simulink model "UKF_liuxg"  (R2017a)
settings: Solver=FixedStepAuto  StartTime=0.0  StopTime=13135  FixedStep=1  RelTol=1e-3
undefined symbols (not defined in the file): sigbuilder_block
libraries: dspmtrx3 x2
settings Model: Creator=HP  LastModifiedBy=HP
settings DataIOCC: ReturnWorkspaceOutputs=on
settings DebuggingCC: UnconnectedInputMsg=none  UnconnectedOutputMsg=none  UnconnectedLineMsg=none
settings ModelReferenceCC: EnableRefExpFcnMdlSchedulingChecks=off
settings SFSimCC: SimUseLocalCustomCode=on
settings RTWCC: RTWUseLocalCustomCode=on

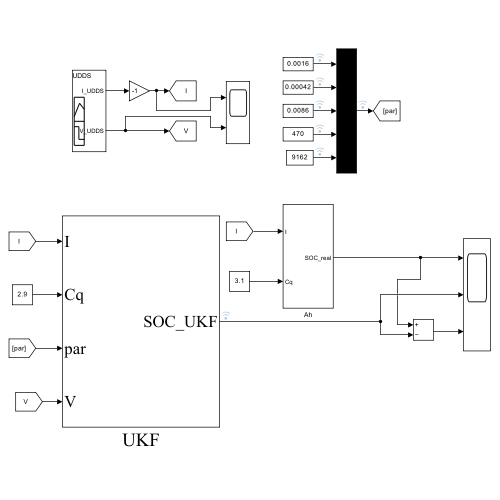
[thumbnail: Simulink's stored preview of the top-level diagram]
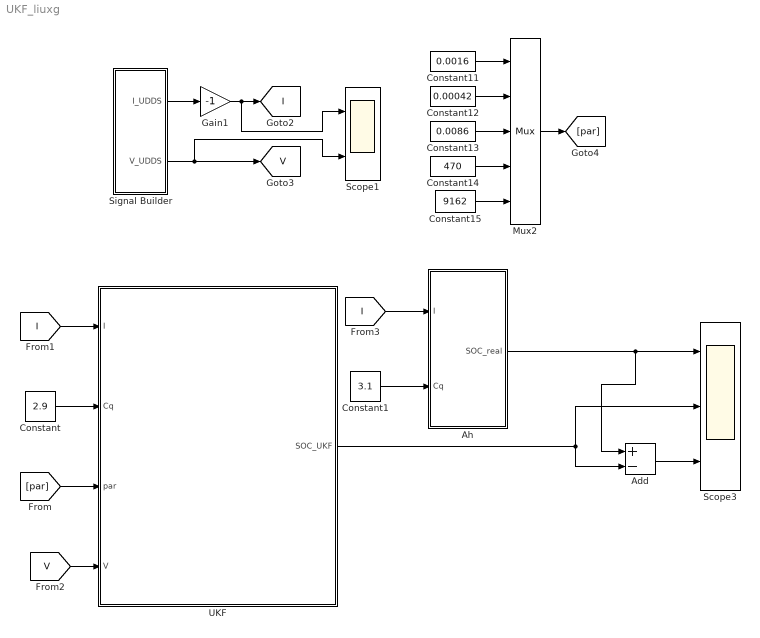
== system UKF_liuxg ==
  Add : Sum  Inputs=+-
  Ah : Subsystem
  Constant : Constant  Value=2.9
  Constant1 : Constant  Value=3.1
  Constant11 : Constant  Value=0.0016
  Constant12 : Constant  Value=0.00042
  Constant13 : Constant  Value=0.0086
  Constant14 : Constant  Value=470
  Constant15 : Constant  Value=9162
  Gain1 : Gain  Gain=-1
  Mux2 : Mux  Inputs=5
  Scope1 : Scope  NumInputPorts=2
  Scope3 : Scope  NumInputPorts=3
  Signal Builder : Subsystem  Tag=STV Subsys  LoadFcn=sigbuilder_block('load');  StartFcn=sigbuilder_block('start');  StopFcn=sigbuilder_block('stop');  ClipboardFcn=sigbuilder_block('clipboard');  mask(Sigbuilder block){tuvar=[0:10]}
      mask init:
      | if ~strcmp(get_param(bdroot(gcb),'SimulationStatus'),'stopped'),tuvar = sigbuilder_block('maskInit'); end
      settings: CopyFcn=sigbuilder_block('copy');  DeleteFcn=sigbuilder_block('delete');  ModelCloseFcn=sigbuilder_block('modelClose');  PreSaveFcn=sigbuilder_block('preSave');  PauseFcn=sigbuilder_block('pause');  ContinueFcn=sigbuilder_block('continue');  NameChangeFcn=sigbuilder_block('namechange');  OpenFcn=sigbuilder_block('open',[0 63 1141.2 523.8 ]);  CloseFcn=sigbuilder_block('close');
      mask Display: plot(0, 0, 100, 100,[2, 2, 32, 32, 2], [68, 8, 8, 68, 68],[32, 2], [38, 38], [32, 19, 2],[53, 60, 44], [32, 17, 17, 2],[16, 16, 31, 31]);txt = getActiveGroup(gcbh);text(2, 100, txt,'verticalAlignment', 'top');
  UKF : Subsystem  mask{Q_UKF=[0.0000000001,0.00001,0.00000001], R_UKF=0.1, X0_UKF=[0.8;0;0], P0_UKF=[0.01,0.01,0.01], f_OCV=[-542.328042776627	3066.57848545083	-7520.83333797876	10535.7804287577	-9327.72222618654	5441.66203885271	-2111.60737486106	536.514433511755	-85.4036277861597	8.01612301618486	2.03460000000008], beta=2, alf=1, ki=0, L=3}
      mask prompts: Q_UKF "系统协方差Q"; R_UKF "测量协方差R"; X0_UKF "状态初始值X0"; P0_UKF "估计协方差初始值P0"; f_OCV "开路电压对SOC的函数"; beta "非负权系数beta"; alf "采样点分布状态参数alf"; ki "无界非待选参数ki"; L "状态维度L"
      mask DialogControl DescGroupVar Prompt: UKF滤波算法
      mask DialogControl ParameterGroupVar Prompt: 滤波参数设置
      mask DialogControl ParameterGroupVar2 Prompt: sigma参数设置
  tag scope: I=global, V=global
  wires:
  Constant15/1 -> Mux2/5
  Constant11/1 -> Mux2/1
  Constant13/1 -> Mux2/3
  Constant14/1 -> Mux2/4
  Constant12/1 -> Mux2/2
  Mux2/1 -> [par]
  Signal Builder/1(I_UDDS) -> Gain1/1
  Signal Builder/2(V_UDDS) -> [V], Scope1/2
  Gain1/1 -> Scope1/1, [I]
  [par] -> UKF/3(par)
  [I] -> UKF/1(I)
  [V] -> UKF/4(V)
  Constant/1 -> UKF/2(Cq)
  UKF/1(SOC_UKF) -> Scope3/2, Add/2
  [I] -> Ah/1(I)
  Constant1/1 -> Ah/2(Cq)
  Ah/1(SOC_real) -> Add/1, Scope3/1
  Add/1 -> Scope3/3

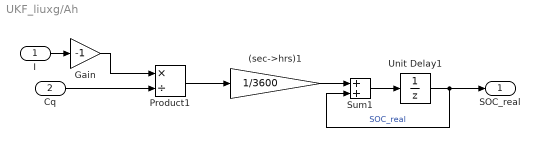
== system UKF_liuxg/Ah ==
  I : Inport
  Cq : Inport  Port=2
  (sec->hrs)1 : Gain  Gain=1/3600  SaturateOnIntegerOverflow=on  OutDataTypeStr=Inherit: Same as input  ParamDataTypeStr=Inherit: Same as input
  Gain : Gain  Gain=-1
  Product1 : Product  Inputs=*/
  Sum1 : Sum
  Unit Delay1 : UnitDelay  InitialCondition=1  SampleTime=-1  HasFrameUpgradeWarning=on
  SOC_real : Outport
  wires:
  I/1 -> Gain/1
  Gain/1 -> Product1/1
  Product1/1 -> (sec->hrs)1/1
  (sec->hrs)1/1 -> Sum1/1
  Unit Delay1/1 -> Sum1/2, SOC_real/1  "SOC_real"
  Sum1/1 -> Unit Delay1/1
  Cq/1 -> Product1/2

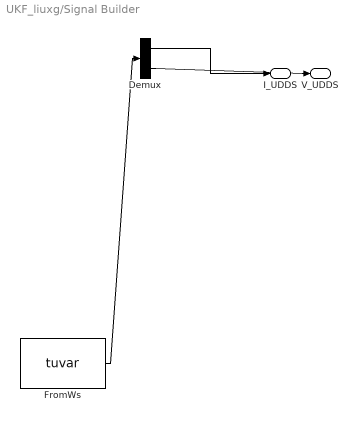
== system UKF_liuxg/Signal Builder ==
  Demux : Demux  Tag=STV Demux  Outputs=2
  FromWs : FromWorkspace  Tag=STV FromWs  VariableName=tuvar
      SigBuilderData=|
      | dataSet.timeRange = [1 13135]
      | dataSet.name = 'UDDS'
      | sbobj.Name = 'Signal Builder'
      | sbobj.Groups.Name = 'UDDS'
      | sbobj.Groups.Signals(1).Name = 'I_UDDS'
      | sbobj.Groups.Signals(1).XData = [1 2 3 4 5 6 7 8 9 10 11 12 ... (13135 elements, 1x13135)]
      | sbobj.Groups.Signals(1).YData = [0 -0.0248 -0.1178 -0.1178 -0.1178 -0.1178 -0.1178 -0.1178 -0.1178 -0.1178 -0.1178 -0.1178 ... (13135 elements, 1x13135)]
      | sbobj.Groups.Signals(2).Name = 'V_UDDS'
      | sbobj.Groups.Signals(2).XData = [1 2 3 4 5 6 7 8 9 10 11 12 ... (13135 elements, 1x13135)]
      | sbobj.Groups.Signals(2).YData = [2.6686 2.6686 2.6683 2.6683 2.6683 2.6677 2.6677 2.6677 2.6677 2.6674 2.6674 2.6674 ... (13135 elements, 1x13135)]
      | sbobj.Groups.TimeRange = [1 9002]
  I_UDDS : Outport  Tag=STV Outport
  V_UDDS : Outport  Tag=STV Outport  Port=2
  wires:
  FromWs/1 -> Demux/1
  Demux/1 -> I_UDDS/1
  Demux/2 -> V_UDDS/1

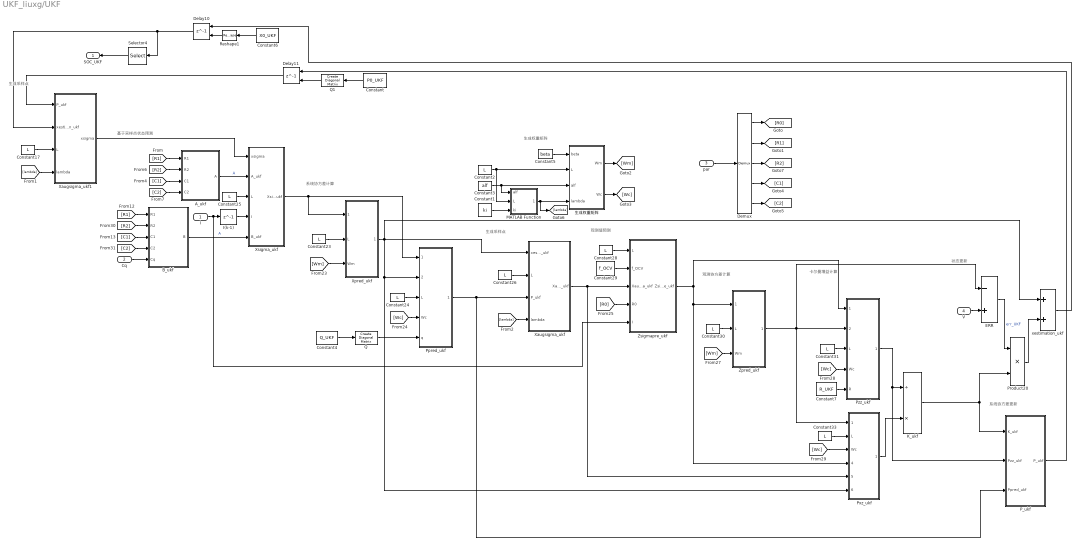
== system UKF_liuxg/UKF ==
  note: 生成权重矩阵
  note: 系统协方差更新
  note: 状态更新
  note: 卡尔曼增益计算
  note: 观测协方差计算
  note: 观测值预测
  note: 生成采样点
  note: 系统协方差计算
  note: 基于采样点状态预测
  note: 生成采样点
  I : Inport
  Cq : Inport  Port=2
  par : Inport  Port=3
  V : Inport  Port=4
  A_ukf : MATLAB Function  TreatAsAtomicUnit=on
  B_ukf : MATLAB Function  TreatAsAtomicUnit=on
  Constant : Constant  Value=P0_UKF
  Constant1 : Constant  Value=ki
  Constant{2,17,23..26,28,30..31,33} (10 alike) : Constant  Value=L
  Constant29 : Constant  Value=f_OCV
  Constant3 : Constant  Value=alf
  Constant4 : Constant  Value=Q_UKF
  Constant5 : Constant  Value=beta
  Constant6 : Constant  Value=X0_UKF
  Constant7 : Constant  Value=R_UKF
  Delay10 : Delay  DelayLength=1  InitialConditionSource=Input port
      settings: InputPortMap=u0,p4
  Delay11 : Delay  DelayLength=1  InitialConditionSource=Input port  InitialCondition=0.001*eye(L)
      settings: InputPortMap=u0,p4
  Demux : Demux  Outputs=5
  ERR : Sum  Inputs=-+
  I(k-1) : Delay  DelayLength=1
  K_ukf : Product  Inputs=/*
  MATLAB Function : MATLAB Function  TreatAsAtomicUnit=on
  P_ukf : MATLAB Function  TreatAsAtomicUnit=on
  Ppred_ukf : MATLAB Function  TreatAsAtomicUnit=on
  Product20 : Product
  Pxz_ukf : MATLAB Function  TreatAsAtomicUnit=on
  Pzz_ukf : MATLAB Function  TreatAsAtomicUnit=on
  Q : dspmtrx3/Create Diagonal Matrix
  Q1 : dspmtrx3/Create Diagonal Matrix
  Reshape1 : Reshape  OutputDimensionality=Customize  OutputDimensions=[3,1]
  Selector4 : Selector  NumberOfDimensions=2  InputPortWidth=3  IndexOptions=Index vector (dialog),Index vector (dialog)  Indices=[1],1  OutputSizes=1,1
  Xaugsigma_ukf : MATLAB Function  TreatAsAtomicUnit=on
  Xaugsigma_ukf1 : MATLAB Function  TreatAsAtomicUnit=on
  Xpred_ukf : MATLAB Function  TreatAsAtomicUnit=on
  Xsigma_ukf : MATLAB Function  TreatAsAtomicUnit=on
  Zpred_ukf : MATLAB Function  TreatAsAtomicUnit=on
  Zsigmapre_ukf : MATLAB Function  TreatAsAtomicUnit=on
  xestimation_ukf : Sum
  生成权重矩阵 : MATLAB Function  TreatAsAtomicUnit=on
  SOC_UKF : Outport
  wires:
  Reshape1/1 -> Delay10/2
  [R0] -> Zsigmapre_ukf/4(R0)
  Q/1 -> Ppred_ukf/5(q)
  P_ukf/1(P_ukf) -> Delay11/1
  Constant17/1 -> Xaugsigma_ukf1/3(L)
  Zsigmapre_ukf/1(Zsigmapre_ukf) -> Pzz_ukf/1(Zsigmapre_ukf), Zpred_ukf/1(Zsigmapre_ukf), Pxz_ukf/4(Zsigmapre_ukf)
  生成权重矩阵/1(Wm) -> [Wm]
  Constant7/1 -> Pzz_ukf/5(R)
  Constant29/1 -> Zsigmapre_ukf/2(f_OCV)
  Zpred_ukf/1(Zpred_ukf) -> Pzz_ukf/2(Zpred_ukf), Pxz_ukf/1(Zpred_ukf), ERR/1
  Xpred_ukf/1(Xpred_ukf) -> Pxz_ukf/6(Xpred_ukf), Ppred_ukf/2(Xpred_ukf), xestimation_ukf/1, Xaugsigma_ukf/1(xestimation_ukf)
  Xsigma_ukf/1(Xsigma_ukf) -> Xpred_ukf/1(Xsigma_ukf), Ppred_ukf/1(Xsigma_ukf)
  Delay11/1 -> Xaugsigma_ukf1/1(P_ukf)
  Ppred_ukf/1(Ppred_ukf) -> P_ukf/3(Ppred_ukf), Xaugsigma_ukf/3(P_ukf)
  Xaugsigma_ukf1/1(xsigma) -> Xsigma_ukf/1(xsigma)
  xestimation_ukf/1 -> Delay10/1
  I(k-1)/1 -> Xsigma_ukf/4(I)
  B_ukf/1(B) -> Xsigma_ukf/5(B_ukf)  "A"
  Constant26/1 -> Xaugsigma_ukf/2(L)
  [lambda] -> Xaugsigma_ukf/4(lambda)
  Delay10/1 -> Xaugsigma_ukf1/2(xestimation_ukf), Selector4/1
  Xaugsigma_ukf/1(Xaugsigma_ukf) -> Zsigmapre_ukf/3(Xaugsigma_ukf), Pxz_ukf/5(Xaugsigma_ukf)
  [R1] -> B_ukf/1(R1)
  [lambda] -> Xaugsigma_ukf1/4(lambda)
  Constant33/1 -> Pxz_ukf/2(L)
  Constant4/1 -> Q/1
  Constant30/1 -> Zpred_ukf/2(L)
  K_ukf/1 -> Product20/2, P_ukf/1(K_ukf)
  Constant28/1 -> Zsigmapre_ukf/1(L)
  [Wm] -> Xpred_ukf/3(Wm)
  生成权重矩阵/2(Wc) -> [Wc]
  Selector4/1 -> SOC_UKF/1
  [Wc] -> Pxz_ukf/3(Wc)
  Constant31/1 -> Pzz_ukf/3(L)
  [Wm] -> Zpred_ukf/3(Wm)
  Constant6/1 -> Reshape1/1
  A_ukf/1(A) -> Xsigma_ukf/2(A_ukf)  "A"
  Product20/1 -> xestimation_ukf/2
  [Wc] -> Pzz_ukf/4(Wc)
  Pzz_ukf/1(Pzz_ukf) -> K_ukf/1, P_ukf/2(Pzz_ukf)
  [Wc] -> Ppred_ukf/4(Wc)
  Pxz_ukf/1(Pxz_ukf) -> K_ukf/2
  Constant24/1 -> Ppred_ukf/3(L)
  V/1 -> ERR/2
  Constant23/1 -> Xpred_ukf/2(L)
  [C1] -> A_ukf/3(C1)
  Constant25/1 -> Xsigma_ukf/3(L)
  [C2] -> B_ukf/4(C2)
  Cq/1 -> B_ukf/5(Cq)
  [R1] -> A_ukf/1(R1)
  [R2] -> A_ukf/2(R2)
  [C2] -> A_ukf/4(C2)
  I/1 -> Zsigmapre_ukf/5(I), I(k-1)/1
  Demux/4 -> [C1]
  Demux/3 -> [R2]
  Demux/1 -> [R0]
  par/1 -> Demux/1
  Demux/5 -> [C2]
  Demux/2 -> [R1]
  [R2] -> B_ukf/2(R2)
  [C1] -> B_ukf/3(C1)
  Constant/1 -> Q1/1
  Q1/1 -> Delay11/2
  Constant5/1 -> 生成权重矩阵/1(beta)
  Constant2/1 -> 生成权重矩阵/2(L), MATLAB Function/2(L)
  Constant3/1 -> 生成权重矩阵/3(alf), MATLAB Function/1(alf)
  MATLAB Function/1(lambda) -> 生成权重矩阵/4(lambda), [lambda]
  Constant1/1 -> MATLAB Function/3(ki)
  ERR/1 -> Product20/1  "err_UKF"

== matlab function UKF_liuxg/UKF/生成权重矩阵 ==
  data: beta input; L input; alf input; lambda input; Wm output size=[7,1]; Wc output size=[7,1]
function [Wm,Wc] = fcn(beta,L,alf,lambda)
Wm=zeros(7,1);
Wc=zeros(7,1);
Wm(1)=lambda/(L+lambda);
Wc(1)=lambda/((L+lambda)+1-alf^2+beta);
for j=2:2*L+1
    Wm(j)=1/(2*(L+lambda));%下标m为均值权重
    Wc(j)=1/(2*(L+lambda));%下标c为协方差权重
end

== matlab function UKF_liuxg/UKF/Xpred_ukf ==
  data: Xsigma_ukf input; Xpred_ukf output; L input; Wm input
function Xpred_ukf  = E(Xsigma_ukf,L,Wm)
Xpred_ukf=zeros(size(Xsigma_ukf,1),1);
for k=1:2*L+1
    Xpred_ukf=Xpred_ukf+Wm(k)*Xsigma_ukf(:,k);
end
end

== matlab function UKF_liuxg/UKF/Ppred_ukf ==
  data: Xsigma_ukf input; Xpred_ukf input; Ppred_ukf output size=[L,L]; L input; Wc input; q input
function Ppred_ukf  = EAE(Xsigma_ukf,Xpred_ukf,L,Wc,q)
Ppred_ukf=zeros(size(Xsigma_ukf,1),size(Xsigma_ukf,1));%协方差预测均值
for k=1:2*L+1
    Ppred_ukf=Ppred_ukf+Wc(k)*(Xsigma_ukf(:,k)-Xpred_ukf)*(Xsigma_ukf(:,k)-Xpred_ukf)';
end
Ppred_ukf=Ppred_ukf+q;
end

== matlab function UKF_liuxg/UKF/Xaugsigma_ukf ==
  data: xestimation_ukf input; L input; Xaugsigma_ukf output size=[L,2*L+1]; P_ukf input; lambda input
function Xaugsigma_ukf = sigma(xestimation_ukf,L,P_ukf,lambda)
cho_ukf=(chol(P_ukf*(L+lambda)))';%cho=chol(X)用于对矩阵X进行Cholesky分解，产生一个上三角cho，使得cho'cho=X，若X为非对称正定，则报错；
XaugsigmaP1_ukf=zeros(size(xestimation_ukf,1),size(xestimation_ukf,1));
XaugsigmaP2_ukf=zeros(size(xestimation_ukf,1),size(xestimation_ukf,1));
for k=1:L
    XaugsigmaP1_ukf(:,k)=xestimation_ukf+cho_ukf(:,k);
    XaugsigmaP2_ukf(:,k)=xestimation_ukf-cho_ukf(:,k);
end
Xaugsigma_ukf=[xestimation_ukf XaugsigmaP1_ukf XaugsigmaP2_ukf];%获得2*L+1个sigma点
end

== matlab function UKF_liuxg/UKF/Zsigmapre_ukf ==
  data: L input; Zsigmapre_ukf output size=[1,2*L+1]; f_OCV input; Xaugsigma_ukf input; R0 input; I input
function Zsigmapre_ukf= err(L,f_OCV,Xaugsigma_ukf,R0,I)
    Zsigmapre_ukf=zeros(1,2*size(Xaugsigma_ukf,1)+1);
    for k=1:2*L+1
        Zsigmapre_ukf(1,k)=polyval(f_OCV,Xaugsigma_ukf(1,k))-Xaugsigma_ukf(2,k)-Xaugsigma_ukf(3,k)-R0*I;
    end
end

== matlab function UKF_liuxg/UKF/Zpred_ukf ==
  data: Zsigmapre_ukf input; Zpred_ukf output; L input; Wm input
function Zpred_ukf  = E(Zsigmapre_ukf,L,Wm)
Zpred_ukf=zeros(size(Zsigmapre_ukf,1),1);
for k=1:2*L+1
    Zpred_ukf=Zpred_ukf+Wm(k)*Zsigmapre_ukf(:,k);
end
end

== matlab function UKF_liuxg/UKF/Pzz_ukf ==
  data: Zsigmapre_ukf input; Zpred_ukf input; Pzz_ukf output size=[1,1]; L input; Wc input; R input
function Pzz_ukf  = EAE(Zsigmapre_ukf,Zpred_ukf,L,Wc,R)
Pzz_ukf=zeros(size(Zsigmapre_ukf,1),size(Zsigmapre_ukf,1));%协方差预测均值
for k=1:2*L+1
    Pzz_ukf=Pzz_ukf+Wc(k)*(Zsigmapre_ukf(:,k)-Zpred_ukf)*(Zsigmapre_ukf(:,k)-Zpred_ukf)';
end
Pzz_ukf=Pzz_ukf+R;
end

== matlab function UKF_liuxg/UKF/Pxz_ukf ==
  data: Zpred_ukf input; L input; Wc input; Zsigmapre_ukf input; Xaugsigma_ukf input; Xpred_ukf input; Pxz_ukf output size=[L,1]
function Pxz_ukf= fcn(Zpred_ukf,L,Wc,Zsigmapre_ukf,Xaugsigma_ukf,Xpred_ukf)
    Pxz_ukf=zeros(size(Xpred_ukf,1),1);
    for k=1:2*L+1
        Pxz_ukf=Pxz_ukf+Wc(k)*(Xaugsigma_ukf(:,k)-Xpred_ukf)*(Zsigmapre_ukf(1,k)-Zpred_ukf)'; 
    end

== matlab function UKF_liuxg/UKF/Xsigma_ukf ==
  data: xsigma input size=[L,2*L+1]; A_ukf input; L input; I input; Xsigma_ukf output size=[L,2*L+1]; B_ukf input
function Xsigma_ukf = pre(xsigma,A_ukf,L,I,B_ukf)
Xsigma_ukf=zeros(size(xsigma,1),2*size(xsigma,1)+1);
for k=1:2*L+1
    Xsigma_ukf(:,k)=A_ukf*xsigma(:,k)+B_ukf*I;
end
end

== matlab function UKF_liuxg/UKF/P_ukf ==
  data: K_ukf input; Pzz_ukf input; Ppred_ukf input; P_ukf output
function P_ukf= fcn(K_ukf,Pzz_ukf,Ppred_ukf)
P_ukf=Ppred_ukf-K_ukf*Pzz_ukf*K_ukf';
end

== matlab function UKF_liuxg/UKF/Xaugsigma_ukf1 ==
  data: P_ukf input; xestimation_ukf input; xsigma output size=[L,2*L+1]; L input; lambda input
function xsigma = sigma(P_ukf,xestimation_ukf,L,lambda)
cho_ukf=(chol(P_ukf*(L+lambda)))';%cho=chol(X)用于对矩阵X进行Cholesky分解，产生一个上三角cho，使得cho'cho=X，若X为非对称正定，则报错；
xgamaP1_ukf=zeros(size(xestimation_ukf,1),size(xestimation_ukf,1));
xgamaP2_ukf=zeros(size(xestimation_ukf,1),size(xestimation_ukf,1));
for k=1:L
    xgamaP1_ukf(:,k)=xestimation_ukf+cho_ukf(:,k);
    xgamaP2_ukf(:,k)=xestimation_ukf-cho_ukf(:,k);
end
xsigma=[xestimation_ukf xgamaP1_ukf xgamaP2_ukf];%获得2*L+1个sigma点
end

== matlab function UKF_liuxg/UKF/A_ukf ==
  data: R1 input; A output; R2 input; C1 input; C2 input
function A = fcn(R1,R2,C1,C2)
tao1=R1*C1;
tao2=R2*C2;
A=[1 0 0;
    0 exp(-1/tao1) 0;
    0 0 exp(-1/tao2)];
end

== matlab function UKF_liuxg/UKF/B_ukf ==
  data: R1 input; B output; R2 input; C1 input; C2 input; Cq input
function B = fcn(R1,R2,C1,C2,Cq)
tao1=R1*C1;
tao2=R2*C2;
B=[-1/(3600*Cq);
    R1*(1-exp(-1/tao1));
    R2*(1-exp(-1/tao2))];
end

== matlab function UKF_liuxg/UKF/MATLAB Function ==
  data: alf input; L input; lambda output; ki input
function lambda= fcn(alf,L,ki)
lambda=alf*alf*(L+ki)-L;
end
